simulink model "Compare_3level"  (R2024b)
settings: Solver=ode1  StartTime=0.0  StopTime=4  FixedStep=Ts  RelTol=1e-3
PreLoadFcn:
  | Net_improve_init;L=Lac_MV;Ts=20e-6;Tctrl=Ts;Rac_MV=1;
PostLoadFcn:
  | Net_improve_init;L=Lac_MV;Ts=20e-6;Tctrl=Ts;Rac_MV=1;
InitFcn:
  | Net_improve_init;L=Lac_MV;Ts=20e-6;Tctrl=Ts;Rac_MV=1;
undefined symbols (not defined in the file or in its folder): C1, dend, DiscIntNeverNeededParam, f_cari, fs, Lac_MV, numd, Pref, R1, Vac_peak_MV, Vdc
libraries: powerlib_extras x15, spsControlledVoltageSourceLib x14, spsIGBTDiodeLib x12, spsCurrentMeasurementLib x8, spsGroundLib x7, spsSeriesRLCBranchLib x7, spsVoltageMeasurementLib x6, spsThreePhaseVIMeasurementLib x5, spsControlledCurrentSourceLib x3, spsIdealSwitchLib x3, spsPower3phInstantaneousLib x3, simulink x3
(part 1 of 2)
Description:
  | The Model initialization function Callback automatically
  | 
  | sets the sample time  to 2e-6 sec.  and loads the initial
  | 
  | states vector xInitial. The initial state vector is saved in the
  | 
  | power_acdrive_init.mat file.
  | 
  | 
  | 
  | Check  the Initial state checkbox in the Simulation
  | 
  | parameters/Workspace I/O to start in steady state with a
  | 
  | speed of 120 rad/s and a torque of 0 N.m/s,
  | 
  | 
  | Copyright 2008-2015 The MathWorks, Inc.
settings Model: Creator=WeiLi  LastModifiedBy=KeXing
settings SolverCC: AlgebraicLoopSolver=TrustRegion
settings DataIOCC: SaveFinalState=on  SaveFormat=Array  SignalLoggingSaveFormat=ModelDataLogs  SaveOutput=off  SaveTime=off  ReturnWorkspaceOutputs=off  SignalLoggingName=sigsOut
settings OptimizationCC: BlockReduction=off  ExpressionDepthLimit=2147483647  InitFltsAndDblsToZero=on  LifeSpan=inf
settings DebuggingCC: SaveWithParameterizedLinksMsg=none  UnderspecifiedInitializationDetection=Classic  MergeDetectMultiDrivingBlocksExec=none  CheckExecutionContextPreStartOutputMsg=on  SignalResolutionControl=TryResolveAllWithWarning  MultiTaskDSMMsg=warning  MultiTaskCondExecSysMsg=none  FcnCallInpInsideContextMsg=warning  UnconnectedInputMsg=warning  UnconnectedLineMsg=warning  StateNameClashWarn=warning  SFUnexpectedBacktrackingDiag=warning  SFNoUnconditionalDefaultTransitionDiag=warning  SFExecutionAtInitializationDiag=none  ArithmeticOperatorsInVariantConditions=warning
settings HardwareCC: ProdBitPerPointer=32  ProdBitPerSizeT=32  ProdBitPerPtrDiffT=32  ProdLargestAtomicFloat=None  ProdIntDivRoundTo=Undefined  ProdEndianess=Unspecified  ProdWordSize=32  ProdHWDeviceType=32-bit Generic  TargetUnknown=on
settings ModelReferenceCC: EnableRefExpFcnMdlSchedulingChecks=on  PropagateSignalLabelsOutOfModel=off
settings SFSimCC: SimUseLocalCustomCode=off  CustomCodeUndefinedFunction=UseInterfaceOnly
settings RTWCC: RTWUseLocalCustomCode=off  GPUComputeCapability=3.5
settings CodeAppCC: StateflowObjectComments=on
settings GRTTargetCC: TargetFcnLib=ansi_tfl_tmw.mat  TargetLangStandard=C89/C90 (ANSI)  CombineOutputUpdateFcns=off  GRTInterface=on
settings ConfigComp: CovMetricSettings=dw  CovSaveCumulativeToWorkspaceVar=on  CovSaveSingleToWorkspaceVar=on  CovExternalEMLEnable=off
settings SimscapeCC: SimscapeNormalizeSystem=off

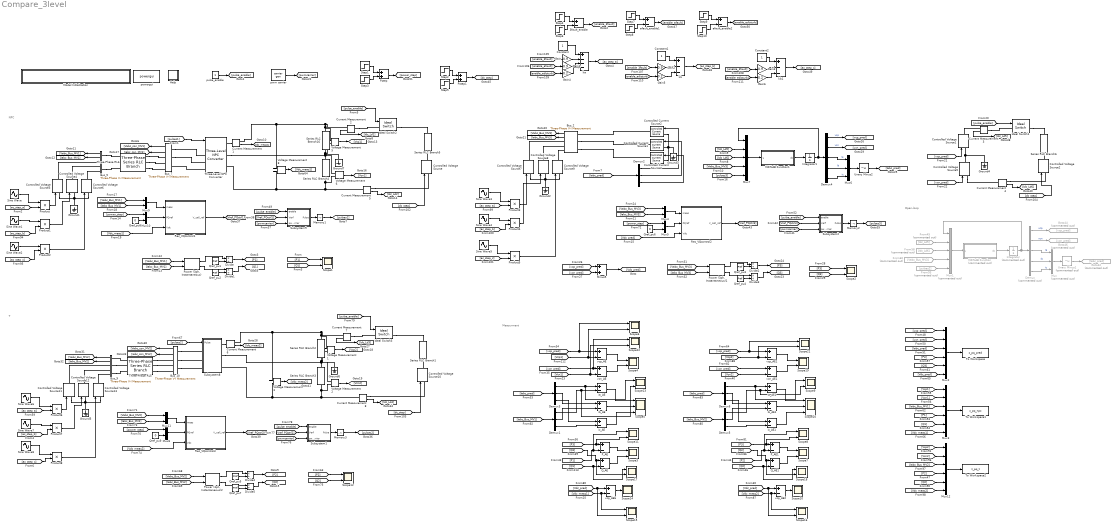
== system Compare_3level ==
  note: NPC
  note: T
  note: Open-loop
  note: Measurment
  3fault_enable : Sum  Inputs=+-
  Bus_{2,5,7,9..10} (5 alike) : spsThreePhaseVIMeasurementLib/Three-Phase V-I Measurement  VoltageMeasurement=phase-to-ground  SetLabelV=off  LabelV=Vabc  Vpu=off  VpuLL=off  CurrentMeasurement=yes  SetLabelI=off  LabelI=Iabc  Ipu=off  Pbase=P_AC  Vbase=V_AC_prim  OutputType=Complex  PhasorSimulation=off  PSBequivalent=0
  Constant : Constant
  Constant1 : Constant
  Constant2 : Constant
  Controlled Current Source1 : spsControlledCurrentSourceLib/Controlled Current Source  Initialize=on  Source_Type=AC  Amplitude=0  Phase=0  Frequency=0  Measurements=None
  Controlled Current Source2 : spsControlledCurrentSourceLib/Controlled Current Source  Initialize=on  Source_Type=AC  Amplitude=0  Phase=0  Frequency=0  Measurements=None
  Controlled Current Source3 : spsControlledCurrentSourceLib/Controlled Current Source  Initialize=on  Source_Type=AC  Amplitude=0  Phase=0  Frequency=0  Measurements=None
  Controlled Voltage Source{,1..2,5,10} (5 alike) : spsControlledVoltageSourceLib/Controlled Voltage Source  Initialize=on  Source_Type=DC  Amplitude=3000  Phase=0  Frequency=0  Measurements=None
  Controlled Voltage Source{3..4,6..9,11..13} (9 alike) : spsControlledVoltageSourceLib/Controlled Voltage Source  Initialize=off  Source_Type=AC  Amplitude=0  Phase=0  Frequency=fs  Measurements=None
  Current Measurement{1..8} (8 alike) : spsCurrentMeasurementLib/Current Measurement  PhasorSimulation=off  OutputType=Complex  PSBequivalent=0
  Demux : Demux  Commented=on  Outputs=5
  Demux{1..3,5..6} (5 alike) : Demux  Outputs=3
  Demux4 : Demux  Outputs=5
  Divide{,1..5} (6 alike) : Product  Inputs=*/
  From45 : From  Commented=on  GotoTag=Idc_Ld5
  From58 : From  Commented=on  GotoTag=Idc_Ld6
  From60 : From  Commented=on  GotoTag=Vabc_Bus_MV3
  From93 : From  Commented=on  GotoTag=pulses2
  Gain{,1..3} (4 alike) : Gain  Gain=0.9
  Gain4 : Gain  Gain=0.2
  Gain5 : Gain  Gain=0.2
  Gain6 : Gain  Gain=0.2
  Goto42 : Goto  Commented=on  GotoTag=Iabc_pred
  Goto44 : Goto  Commented=on  GotoTag=vcp_pred
  Goto46 : Goto  Commented=on  GotoTag=vcn_pred
  Ground{1..7} (7 alike) : spsGroundLib/Ground  LConnTagsString=a
  Help : Subsystem  mask(OpDoc){docfile=../Help/help.html}
      mask init:
      | %patch([1,1,0,0,.8,1],[.8,0,0,1,1,.8],[.8 .8 .8]);
      | %patch([.15 .78 .78 .15 .15],[.8 .8 .83 .83 .8],[.9 .9 .9]);
      | %patch([.15 .78 .78 .15 .15],[.7 .7 .73 .73 .8],[.9 .9 .9]);
      | %patch([.15 .78 .78 .15 .15],[.6 .6 .63 .63 .6],[.9 .9 .9]);
      | %patch([.15 .78 .78 .15 .15],[.5 .5 .53 .53 .5],[.9 .9 .9]);
      | %patch([.15 .78 .78 .15 .15],[.4 .4 .43 .43 .4],[.9 .9 .9]);
      settings: OpenFcn=OpHelp_cb(gcb);
      mask Display: image(imread('opdoc.bmp'))
  Ideal Switch1 : spsIdealSwitchLib/Ideal Switch  Ron=0.001  Lon=0  IC=0  Rs=1e9  Cs=inf  Measurements=on
  Ideal Switch2 : spsIdealSwitchLib/Ideal Switch  Ron=0.001  Lon=0  IC=0  Rs=1e9  Cs=inf  Measurements=on
  Ideal Switch3 : spsIdealSwitchLib/Ideal Switch  Ron=0.001  Lon=0  IC=0  Rs=1e9  Cs=inf  Measurements=on
  Integrator : Integrator  Commented=on
  Integrator1 : Integrator
  MATLAB Function : MATLAB Function  Commented=on  TreatAsAtomicUnit=on
  MATLAB Function1 : MATLAB Function  TreatAsAtomicUnit=on
  Memory1 : Memory
  Memory2 : Memory
  Memory3 : Memory
  Minus5 : Sum
  Model Initialization : Subsystem  mask(Model Functions){InitFcnX=Net_improve_init;L=Lac_MV;Ts=20e-6;Tctrl=Ts;Rac_MV=1;, prel=on, posl=on, inif=on, strf=off}
      mask prompts: InitFcnX "Initialisation"; prel "Preload Function"; posl "PostLoad Function"; inif "InitFcn"; strf "StartFcn"
      mask init:
      | currentBlock = gcb;
      | root = bdroot(currentBlock);
      | 
      | if ~strcmp(get_param(root,'BlockDiagramType'),'library')
      |     if prel==1
      |         set_param(root, 'PreLoadFcn', InitFcnX);
      |     else
      |         set_param(root, 'PreLoadFcn', '');
      |     end
      |     if inif==1
      |         set_param(root, 'InitFcn', InitFcnX);
      |     else
      |         set_param(root, 'InitFcn', '');
      |     end
      |     if strf==1
      |         set_param(root, 'StartFcn', InitFcnX);
      |     else
      |         set_param(root, 'StartFcn', '');
      |     end
      |     if posl==1
      |         set_param(root, 'PostLoadFcn', InitFcnX);
      |     else
      |         set_param(root, 'PostLoadFcn', '');
      |     end
      | end
      | 
      | pos = get_param(currentBlock, 'Position');
      | width = pos(3) - pos(1); height = pos(4) - pos(2);
      | txt = [ upper(root) '\n' '- InitFcn. . . . . '  get_param(root, 'InitFcn') ];
      settings: CopyFcn=set_param(gcb,'LinkStatus','none')
      mask Display: text(5, height*0.5, txt, 'horizontalAlignment', 'left', 'verticalAlignment', 'middle') ;
  Mux : Mux  Commented=on  Inputs=3
  Mux1 : Mux  Commented=on  Inputs=5
  Mux{4..5,8..11} (6 alike) : Mux  Inputs=2
  Mux12 : Mux  Inputs=6
  Mux2 : Mux  Inputs=6
  Mux3 : Mux  Inputs=6
  Mux6 : Mux  Inputs=3
  Mux7 : Mux  Inputs=5
  P_AE : Sum  Inputs=+-
  P_AE1 : Sum  Inputs=+-
  "Power (3ph, Instantaneous)" : spsPower3phInstantaneousLib/Power (3ph, Instantaneous)
  "Power (3ph, Instantaneous)1" : spsPower3phInstantaneousLib/Power (3ph, Instantaneous)
  "Power (3ph, Instantaneous)2" : spsPower3phInstantaneousLib/Power (3ph, Instantaneous)
  Product{,1..8} (9 alike) : Product
  Pstep : Sum
  Pstep1 : Sum
  Q_AE : Sum  Inputs=+-
  Q_AE1 : Sum  Inputs=+-
  Qref_pu{1..5,7} (6 alike) : Constant  Value=Pref
  Qref_pu6 : Constant  Value=0
  Qref_pu8 : Constant  Value=0
  Qref_pu9 : Constant  Value=0
  Rec_VQcontrol1 : Subsystem  mask(converter controller){cm=off, base=[Pref, Vac_peak_MV*sqrt(3/2), Vdc/2, fs], LRx=[Lac_MV, Rac_MV], LRx_inpu=off, Kd=[0.3  2]*10/6  %was [1 0.1]   ; [0.1  1]*1, Kp=[0.3 1]*1     %was [1 0.1]   ; [0.1  1]*1, Kvdc=[2 10]*1;   %was [0.5 1]*20 for Cdc=320uF, Vabc_lim=[-1 1], limitVdq=1.1, nadv=6, xtrIctrl1=[0.4 10 10 -10], Ts=Tctrl}
      mask prompts: cm "control mode (check VQ/uncheck PQ), only one terminal in VQ mode"; base "base value for power(VA), ac voltage(V), dc voltage to ground(V), and frequenvy(Hz) [Sb, Vb, Vdcb,freq]"; LRx "commutation inductance and resistance [Lx, Rx]"; LRx_inpu "[Lx, Rx] in pu if checked/ SI unchecked"; Kd "Kp Ki for d-axis PI control [kp ki]"; Kp "Kp Ki for q-axis PI control [kp ki]"; Kvdc "Kp Ki for Vdc PI control [kp ki]"; Vabc_lim "output Vabc limit [min max]"; limitVdq "limit for Vd,Vq (pu, default = 1.1)"; nadv "nb of time step to compesate for delay (default=1)"; xtrIctrl1 "[kp, kp, limitmax, limitmin] for current control (default=[0.4, 10, 10, -10])"
      mask help:
      | input 1, 6 dimentions, Vabc, Iabc, (SI)
      | input 2, 2 dimentions, Pref, Qref (PU)
      | input 3, 6 dimentions, Vcap at up arm a, lower arm a, up arm b, lower arm b, up arm c and lower arm c.
      | input 4, 1 dimention, pulse on
      | input 5, 1 dimention
      |
      | power or current directions: to go into grid is positive
      mask init:
      | if cm==0;
      |     x=['PQ\nmode'];
      | else
      |     x=['VQ\nmode'];
      | end
      | 
      | Sb=base(1);            %VA 3phase power base;
      | Vb=base(2);       %V, line-line rms voltage base
      | Ib=Sb/(sqrt(3)*Vb); %A, rms current base
      | Zb=Vb^2/Sb ;        %ohm, impedence base
      | Vdc=base(3);      %V Vdc+ to ground or ground to Vdc- 
      | frq=base(4);
      | 
      | if LRx_inpu
      |     Rxpu=LRx(2);
      |     Lxpu=LRx(1);
      | else
      |     Rxpu=LRx(2)/Zb;
      |     Lxpu=LRx(1)*2*pi*frq/Zb;
      | end;
      | 
      | ks=Vdc*sqrt(3/2)/Vb;     % ma=1/ks for 1pu dc ->1pu ac;
      | 
      | Kp=Kd;
      mask DialogControl ParameterTabVar0 Prompt: parameters
      mask DialogControl ParameterTabVar01 Prompt: advanced
      mask Display: disp (x);
  Rec_VQcontrol2 : Subsystem  mask(converter controller){cm=off, base=[Pref, Vac_peak_MV*sqrt(3/2), Vdc/2, fs], LRx=[Lac_MV, Rac_MV], LRx_inpu=off, Kd=[0.3  2]*10/6  %was [1 0.1]   ; [0.1  1]*1, Kp=[0.3 1]*1     %was [1 0.1]   ; [0.1  1]*1, Kvdc=[2 10]*1;   %was [0.5 1]*20 for Cdc=320uF, Vabc_lim=[-1 1], limitVdq=1.1, nadv=6, xtrIctrl1=[0.4 10 10 -10], Ts=Tctrl}
      mask prompts: cm "control mode (check VQ/uncheck PQ), only one terminal in VQ mode"; base "base value for power(VA), ac voltage(V), dc voltage to ground(V), and frequenvy(Hz) [Sb, Vb, Vdcb,freq]"; LRx "commutation inductance and resistance [Lx, Rx]"; LRx_inpu "[Lx, Rx] in pu if checked/ SI unchecked"; Kd "Kp Ki for d-axis PI control [kp ki]"; Kp "Kp Ki for q-axis PI control [kp ki]"; Kvdc "Kp Ki for Vdc PI control [kp ki]"; Vabc_lim "output Vabc limit [min max]"; limitVdq "limit for Vd,Vq (pu, default = 1.1)"; nadv "nb of time step to compesate for delay (default=1)"; xtrIctrl1 "[kp, kp, limitmax, limitmin] for current control (default=[0.4, 10, 10, -10])"
      mask help:
      | input 1, 6 dimentions, Vabc, Iabc, (SI)
      | input 2, 2 dimentions, Pref, Qref (PU)
      | input 3, 6 dimentions, Vcap at up arm a, lower arm a, up arm b, lower arm b, up arm c and lower arm c.
      | input 4, 1 dimention, pulse on
      | input 5, 1 dimention
      |
      | power or current directions: to go into grid is positive
      mask init: same as Compare_3level/Rec_VQcontrol1
      mask DialogControl ParameterTabVar0 Prompt: parameters
      mask DialogControl ParameterTabVar01 Prompt: advanced
      mask Display: disp (x);
  Rec_VQcontrol3 : Subsystem  mask(converter controller){cm=off, base=[Pref, Vac_peak_MV*sqrt(3/2), Vdc/2, fs], LRx=[Lac_MV, Rac_MV], LRx_inpu=off, Kd=[0.3  2]*10/6  %was [1 0.1]   ; [0.1  1]*1, Kp=[0.3 1]*1     %was [1 0.1]   ; [0.1  1]*1, Kvdc=[2 10]*1;   %was [0.5 1]*20 for Cdc=320uF, Vabc_lim=[-1 1], limitVdq=1.1, nadv=6, xtrIctrl1=[0.4 10 10 -10], Ts=Tctrl}
      mask prompts: cm "control mode (check VQ/uncheck PQ), only one terminal in VQ mode"; base "base value for power(VA), ac voltage(V), dc voltage to ground(V), and frequenvy(Hz) [Sb, Vb, Vdcb,freq]"; LRx "commutation inductance and resistance [Lx, Rx]"; LRx_inpu "[Lx, Rx] in pu if checked/ SI unchecked"; Kd "Kp Ki for d-axis PI control [kp ki]"; Kp "Kp Ki for q-axis PI control [kp ki]"; Kvdc "Kp Ki for Vdc PI control [kp ki]"; Vabc_lim "output Vabc limit [min max]"; limitVdq "limit for Vd,Vq (pu, default = 1.1)"; nadv "nb of time step to compesate for delay (default=1)"; xtrIctrl1 "[kp, kp, limitmax, limitmin] for current control (default=[0.4, 10, 10, -10])"
      mask help:
      | input 1, 6 dimentions, Vabc, Iabc, (SI)
      | input 2, 2 dimentions, Pref, Qref (PU)
      | input 3, 6 dimentions, Vcap at up arm a, lower arm a, up arm b, lower arm b, up arm c and lower arm c.
      | input 4, 1 dimention, pulse on
      | input 5, 1 dimention
      |
      | power or current directions: to go into grid is positive
      mask init: same as Compare_3level/Rec_VQcontrol1
      mask DialogControl ParameterTabVar0 Prompt: parameters
      mask DialogControl ParameterTabVar01 Prompt: advanced
      mask Display: disp (x);
  Scope{1..4,6..9,11..13,15..19,21..22} (18 alike) : Scope  NumInputPorts=2
  Scope10 : Scope
  Scope14 : Scope
  Scope20 : Scope  NumInputPorts=3
  Scope5 : Scope  NumInputPorts=3
  Series RLC Branch1 : spsSeriesRLCBranchLib/Series RLC Branch  LConnTagsString=__new0  RConnTagsString=__new0  BranchType=R  Resistance=3e3^2/(Pref)/10*2  Inductance=1e-3  SetiL0=off  InitialCurrent=0  Capacitance=C1  Setx0=off  InitialVoltage=0  Measurements=None
  Series RLC Branch{2..4,16} (4 alike) : spsSeriesRLCBranchLib/Series RLC Branch  LConnTagsString=__new0  RConnTagsString=__new0  BranchType=C  Resistance=R1  Inductance=1e-3  SetiL0=off  InitialCurrent=0  Capacitance=C1  Setx0=off  InitialVoltage=0  Measurements=None
  Series RLC Branch5 : spsSeriesRLCBranchLib/Series RLC Branch  LConnTagsString=__new0  RConnTagsString=__new0  BranchType=R  Resistance=3e3^2/(Pref)/10*2  Inductance=1e-3  SetiL0=off  InitialCurrent=0  Capacitance=C1  Setx0=off  InitialVoltage=0  Measurements=None
  Series RLC Branch6 : spsSeriesRLCBranchLib/Series RLC Branch  LConnTagsString=__new0  RConnTagsString=__new0  BranchType=R  Resistance=3e3^2/(Pref)/10*2  Inductance=1e-3  SetiL0=off  InitialCurrent=0  Capacitance=C1  Setx0=off  InitialVoltage=0  Measurements=None
  Sine Wave : Sin  Amplitude=3e3/2*sqrt(2/3)  Frequency=2*pi*fs  SampleTime=0
  Sine Wave1 : Sin  Amplitude=3e3/2*sqrt(2/3)  Frequency=2*pi*fs  Phase=-2*pi/3  SampleTime=0
  Sine Wave2 : Sin  Amplitude=3e3/2*sqrt(2/3)  Frequency=2*pi*fs  Phase=+2*pi/3  SampleTime=0
  Sine Wave3 : Sin  Amplitude=3e3/2*sqrt(2/3)  Frequency=2*pi*fs  SampleTime=0
  Sine Wave4 : Sin  Amplitude=3e3/2*sqrt(2/3)  Frequency=2*pi*fs  Phase=-2*pi/3  SampleTime=0
  Sine Wave5 : Sin  Amplitude=3e3/2*sqrt(2/3)  Frequency=2*pi*fs  Phase=+2*pi/3  SampleTime=0
  Sine Wave6 : Sin  Amplitude=3e3/2*sqrt(2/3)  Frequency=2*pi*fs  SampleTime=0
  Sine Wave7 : Sin  Amplitude=3e3/2*sqrt(2/3)  Frequency=2*pi*fs  Phase=-2*pi/3  SampleTime=0
  Sine Wave8 : Sin  Amplitude=3e3/2*sqrt(2/3)  Frequency=2*pi*fs  Phase=+2*pi/3  SampleTime=0
  Step1 : Step  Time=2.75  Before=-0.8  After=-0.6  SampleTime=0
  Step10 : Step  Time=3.85  SampleTime=0
  Step2 : Step  Time=3.25  Before=3000  After=2400  SampleTime=0
  Step3 : Step  Time=3.0  Before=0.0  After=-0.2  SampleTime=0
  Step4 : Step  Time=1.75  SampleTime=0
  Step5 : Step  Time=3.5  After=600  SampleTime=0
  Step6 : Step  Time=1.9  SampleTime=0
  Step7 : Step  Time=2.5  SampleTime=0
  Step8 : Step  Time=2.65  SampleTime=0
  Step9 : Step  Time=3.70  SampleTime=0
  Subsystem1 : Subsystem
  Subsystem2 : Subsystem
  Subsystem8 : Subsystem
  Subsystem9 : Subsystem
  Three-Level NPC Converter : spsThreeLevelNPCConverterLib/Three-Level NPC Converter  ModelType=Switching devices  Ron=IGBT_Ron  Rs=1e5  Cs=IGBT_Cs  Vforward=[0,0]  Ron_Diode=1e-3  Rs_Diode=1e6  Cs_Diode=inf  Vf_Diode=1e-3  Rs_CurrentSource=inf  Ron_ACsource=1e-3
      settings: LibrarySourceBlock=|
      | sps_lib/Power Electronics/Three-Level
      | NPC Converter
  Three-Phase RL3 : spsThreePhaseSeriesRLCBranchLib/Three-Phase Series RLC Branch  LConnTagsString=A|B|C  RConnTagsString=A|B|C  BranchType=RL  Resistance=Rac_MV  Inductance=Lac_MV  Capacitance=1e-6  Measurements=None
  Three-Phase RL5 : spsThreePhaseSeriesRLCBranchLib/Three-Phase Series RLC Branch  LConnTagsString=A|B|C  RConnTagsString=A|B|C  BranchType=RL  Resistance=Rac_MV  Inductance=Lac_MV  Capacitance=1e-6  Measurements=None
  To Workspace : ToWorkspace  VariableName=z_pq_pred  SampleTime=-1
      settings: Save2DSignal=2-D array (concatenate along first dimension)
  To Workspace1 : ToWorkspace  VariableName=z_pq_npc  SampleTime=-1
      settings: Save2DSignal=2-D array (concatenate along first dimension)
  To Workspace2 : ToWorkspace  VariableName=z_pq_t  SampleTime=-1
      settings: Save2DSignal=2-D array (concatenate along first dimension)
  Unary Minus1 : UnaryMinus  Commented=on
  Unary Minus2 : UnaryMinus
  Voltage Measurement{1..3,5..6,8} (6 alike) : spsVoltageMeasurementLib/Voltage Measurement  PhasorSimulation=off  OutputType=Complex  PSBequivalent=0
  afault_enable1 : Sum  Inputs=+-
  afault_enable2 : Sum  Inputs=+-
  ia_AE : Sum  Inputs=+-
  ia_AE1 : Sum  Inputs=+-
  ib_AE : Sum  Inputs=+-
  ib_AE1 : Sum  Inputs=+-
  ic_AE : Sum  Inputs=+-
  ic_AE1 : Sum  Inputs=+-
  ka : Sum  Inputs=+---
  kb : Sum  Inputs=+--
  kb1 : Sum  Inputs=+--
  powergui : spspowerguiLib/powergui  Priority=2  SimulationMode=Discrete  SampleTime=Ts  frequency=60  Iterations=50  frequencyindice=0  Pbase=100e6  ErrMax=1e-4  UnitsV=kV  UnitsW=MW  buscounter=0  FunctionMessages=off  echomessages=off  EnableUseOfTLC=off  CurrentSourceSwitches=off  DisableSnubberDevices=off  DisableRonSwitches=off  DisableVfSwitches=off  DisplayEquations=off  AutomaticDiscreteSolvers=off  SolverType=Backward Euler  Interpol=off  ExternalGateDelay=off  methode=off  Ts=0  x0status=blocks  SPID=off  SwTol=0  HookPort=off  NonlinearTolerance=1e-4  nMaxIteration=100  ContinueOnMaxIteration=off  RestoreLinks=warning  ResistiveCurrentMeasurement=off  Frange=[0:2:500]  Ylog=off  Xlog=on  ShowGrid=off  save=off  variable=ZData  structure=VI  ZoomFFT=off  StartTime=9  cycles=10  DisplayStyle=2  fundamental=300/pi  FreqAxis=off  MaxFrequency=1000  frequencyindicesteady=1  RmsSteady=1  display=off
  pulse_enable : Constant
  pwm carrier : libMMCcpuv2/carrier gen  fc=f_cari*2  range=[1 0]  Ms=3  Ns=1
  vcn_AE : Sum  Inputs=+-
  vcn_AE1 : Sum  Inputs=+-
  vcp_AE{,1..2,6} (4 alike) : Sum  Inputs=+-
  wires:
  Bus_7/1 -> [Vabc_con_MV1]
  Bus_5/1 -> [Vabc_Bus_MV1]
  Bus_5/2 -> [Iabc_Bus_MV1]
  [pulses1] -> Three-Level NPC Converter/1
  [pulses2] -> Subsystem8/1(Pulse)
  Bus_9/1 -> [Vabc_Bus_MV2]
  Bus_9/2 -> [Iabc_Bus_MV2]
  Bus_10/1 -> [Vabc_con_MV2]
  pwm carrier/1 -> [pwmcarrier]
  pulse_enable/1 -> [pulse_enable]
  [ac_step_c] -> Product2/2
  Sine Wave1/1 -> Product1/1
  [ac_step_a] -> Product/2
  Product2/1 -> Controlled Voltage Source6/1
  Product/1 -> Controlled Voltage Source3/1
  Sine Wave/1 -> Product/1
  Sine Wave2/1 -> Product2/1
  Product1/1 -> Controlled Voltage Source4/1
  [ac_step_b] -> Product1/2
  Bus_7/2 -> [iabc_con_MV1]
  [pwmcarrier] -> Subsystem9/3(pwmcarrier)
  [Iabc_Bus_MV1] -> Mux9/2
  [Vabc_Bus_MV1] -> "Power (3ph, Instantaneous)"/1
  [P1] -> Scope1/1
  [Vref_PQctrl1] -> Subsystem9/2(Verf)
  [Vdc_meas1] -> Rec_VQcontrol1/3(Vdc)
  Qref_pu8/1 -> Mux10/2
  Qref_pu1/1 -> Divide/2
  [Vabc_Bus_MV1] -> Mux9/1
  Mux9/1 -> Rec_VQcontrol1/1(meas)
  [pulse_enable] -> Subsystem9/1(enable)
  [power_step] -> Mux10/1
  Subsystem9/1(Pulse) -> Memory1/1
  Rec_VQcontrol1/1(V_cell_ref) -> [Vref_PQctrl1]
  Divide/1 -> [P1]
  Qref_pu2/1 -> Divide1/2
  Mux10/1 -> Rec_VQcontrol1/2(PQref)
  [Iabc_Bus_MV1] -> "Power (3ph, Instantaneous)"/2
  Divide1/1 -> [Q1]
  "Power (3ph, Instantaneous)"/2 -> Divide1/1
  [Q1] -> Scope1/2
  Memory1/1 -> [pulses1]
  "Power (3ph, Instantaneous)"/1 -> Divide/1
  Voltage Measurement8/1 -> [Vdc_meas1]
  Current Measurement2/1 -> [Idc_Ld1]
  Voltage Measurement6/1 -> [Vcn1]
  Current Measurement5/1 -> [Idc_Ld2]
  [pulse_enable] -> Ideal Switch2/1
  [dc_step] -> Controlled Voltage Source/1
  Current Measurement1/1 -> [Idc_meas1]
  Voltage Measurement5/1 -> [Vcp1]
  [ac_step_b] -> Product7/2
  Sine Wave7/1 -> Product7/1
  Product7/1 -> Controlled Voltage Source12/1
  Sine Wave6/1 -> Product6/1
  Sine Wave8/1 -> Product8/1
  [ac_step_a] -> Product6/2
  [ac_step_c] -> Product8/2
  Product8/1 -> Controlled Voltage Source13/1
  Product6/1 -> Controlled Voltage Source11/1
  Bus_10/2 -> [iabc_con_MV2]
  [power_step] -> Mux8/1
  "Power (3ph, Instantaneous)2"/2 -> Divide5/1
  Qref_pu9/1 -> Mux8/2
  [Vabc_Bus_MV2] -> "Power (3ph, Instantaneous)2"/1
  [Iabc_Bus_MV2] -> "Power (3ph, Instantaneous)2"/2
  Subsystem1/1(Pulse) -> Memory3/1
  [Iabc_Bus_MV2] -> Mux11/2
  Memory3/1 -> [pulses2]
  Qref_pu5/1 -> Divide4/2
  Rec_VQcontrol3/1(V_cell_ref) -> [Vref_PQctrl2]
  Qref_pu7/1 -> Divide5/2
  [Vabc_Bus_MV2] -> Mux11/1
  [pwmcarrier] -> Subsystem1/3(pwmcarrier)
  [pulse_enable] -> Subsystem1/1(enable)
  "Power (3ph, Instantaneous)2"/1 -> Divide4/1
  Divide4/1 -> [P2]
  [Q2] -> Scope12/2
  Mux11/1 -> Rec_VQcontrol3/1(meas)
  [Vref_PQctrl2] -> Subsystem1/2(Verf)
  Mux8/1 -> Rec_VQcontrol3/2(PQref)
  Divide5/1 -> [Q2]
  [P2] -> Scope12/1
  [Vdc_meas2] -> Rec_VQcontrol3/3(Vdc)
  Voltage Measurement2/1 -> [Vcn2]
  Current Measurement6/1 -> [Idc_meas2]
  Current Measurement8/1 -> [Idc_Ld4]
  Current Measurement7/1 -> [Idc_Ld3]
  [dc_step] -> Controlled Voltage Source10/1
  Voltage Measurement1/1 -> [Vcp2]
  Voltage Measurement3/1 -> [Vdc_meas2]
  [pulse_enable] -> Ideal Switch3/1
  [enable_afault] -> Gain1/1
  [enable_edisturb] -> Gain4/1
  Step7/1 -> afault_enable1/1
  afault_enable2/1 -> [enable_edisturb]
  Step5/1 -> Pstep1/2
  Constant/1 -> ka/1
  Gain4/1 -> ka/4
  Gain3/1 -> kb1/2
  Step3/1 -> Pstep/2
  Step6/1 -> 3fault_enable/2
  kb/1 -> [ac_step_b]
  Pstep1/1 -> [dc_step]
  Step10/1 -> afault_enable2/2
  Step4/1 -> 3fault_enable/1
  afault_enable1/1 -> [enable_afault]
  [enable_3fault] -> Gain/1
  Gain6/1 -> kb1/3
  ka/1 -> [ac_step_a]
  Gain1/1 -> ka/3
  [enable_edisturb] -> Gain5/1
  kb1/1 -> [ac_step_c]
  Gain5/1 -> kb/3
  Step2/1 -> Pstep1/1
  [enable_3fault] -> Gain3/1
  Gain2/1 -> kb/2
  3fault_enable/1 -> [enable_3fault]
  Constant1/1 -> kb/1
  [enable_edisturb] -> Gain6/1
  Step9/1 -> afault_enable2/1
  Step8/1 -> afault_enable1/2
  Constant2/1 -> kb1/1
  Step1/1 -> Pstep/1
  Gain/1 -> ka/2
  Pstep/1 -> [power_step]
  [enable_3fault] -> Gain2/1
  [Iabc_pred] -> Demux2/1
  Bus_2/2 -> [Iabc_Bus_MV3]
  Product3/1 -> Controlled Voltage Source7/1
  Demux2/2 -> Controlled Current Source1/1
  [vcp_pred] -> Minus5/1
  Sine Wave3/1 -> Product3/1
  Minus5/1 -> [Vdc_pred]
  [ac_step_a] -> Product3/2
  Sine Wave4/1 -> Product4/1
  Demux2/1 -> Controlled Current Source2/1
  Demux2/3 -> Controlled Current Source3/1
  Sine Wave5/1 -> Product5/1
  Product5/1 -> Controlled Voltage Source9/1
  [ac_step_b] -> Product4/2
  [vcn_pred] -> Minus5/2
  Bus_2/1 -> [Vabc_Bus_MV3]
  [ac_step_c] -> Product5/2
  Product4/1 -> Controlled Voltage Source8/1
  Qref_pu4/1 -> Divide3/2
  "Power (3ph, Instantaneous)1"/1 -> Divide2/1
  [Iabc_Bus_MV3] -> "Power (3ph, Instantaneous)1"/2
  Divide2/1 -> [P3]
  "Power (3ph, Instantaneous)1"/2 -> Divide3/1
  Divide3/1 -> [Q3]
  [Vabc_Bus_MV3] -> "Power (3ph, Instantaneous)1"/1
  Qref_pu3/1 -> Divide2/2
  [Vdc_pred] -> Rec_VQcontrol2/3(Vdc)
  Rec_VQcontrol2/1(V_cell_ref) -> [Vref_PQctrl3]
  [Iabc_Bus_MV3] -> Mux4/2
  Mux5/1 -> Rec_VQcontrol2/2(PQref)
  Qref_pu6/1 -> Mux5/2
  [power_step] -> Mux5/1
  Mux4/1 -> Rec_VQcontrol2/1(meas)
  [Vabc_Bus_MV3] -> Mux4/1
  [Vref_PQctrl3] -> Subsystem2/2(Verf)
  [pulse_enable] -> Subsystem2/1(enable)
  [pwmcarrier] -> Subsystem2/3(pwmcarrier)
  Memory2/1 -> [pulses3]
  Subsystem2/1(Pulse) -> Memory2/1
  Demux4/4 -> Mux6/2  "ib"
  Demux4/5 -> Mux6/3  "ic"
  [Vabc_Bus_MV3] -> Mux7/4
  Mux7/1 -> MATLAB Function1/1(u)
  Demux4/2 -> [vcn_pred]  "vcn"
  [pulses3] -> Mux7/5
  Mux6/1 -> Unary Minus2/1
  [Idc_Ld6] -> Mux7/3
  Demux4/3 -> Mux6/1  "ia"
  Integrator1/1 -> Mux7/1, Demux4/1
  Demux4/1 -> [vcp_pred]  "vcp"
  Unary Minus2/1 -> [Iabc_pred]
  [Idc_Ld5] -> Mux7/2
  MATLAB Function1/1(dz) -> Integrator1/1
  Current Measurement3/1 -> [Idc_Ld5]
  [pulse_enable] -> Ideal Switch1/1
  Current Measurement4/1 -> [Idc_Ld6]
  [vcn_pred] -> Controlled Voltage Source5/1
  [vcp_pred] -> Controlled Voltage Source1/1
  [dc_step] -> Controlled Voltage Source2/1
  Demux/5 -> Mux/3  "ic"
  Demux/1 -> Goto44/1  "vcp"
  Demux/4 -> Mux/2  "ib"
  MATLAB Function/1(dz) -> Integrator/1
  From60/1 -> Mux1/4
  Mux1/1 -> MATLAB Function/1(u)
  From93/1 -> Mux1/5
  Demux/2 -> Goto46/1  "vcn"
  From58/1 -> Mux1/3
  Integrator/1 -> Mux1/1, Demux/1
  Demux/3 -> Mux/1  "ia"
  Mux/1 -> Unary Minus1/1
  Unary Minus1/1 -> Goto42/1
  From45/1 -> Mux1/2
  [Q3] -> Scope2/2
  [P3] -> Scope2/1
  [Vdc_meas2] -> Scope16/1, vcp_AE2/2
  [vcp_pred] -> Mux2/1
  vcn_AE/1 -> Scope4/2
  [Vcp2] -> Scope21/2, vcp_AE1/2
  [Q3] -> Scope18/2, Q_AE1/1
  [Iabc_Bus_MV2] -> Demux5/1
  [Q2] -> Scope18/1, Q_AE1/2
  [Vdc_pred] -> Scope15/2, vcp_AE6/1
  [Vcp1] -> Scope6/2, vcp_AE/2
  vcp_AE/1 -> Scope4/1
  vcp_AE1/1 -> Scope19/1
  Q_AE1/1 -> Scope7/2
  [vcn_pred] -> Mux2/2
  [P3] -> Mux2/4
  Demux1/3 -> ic_AE/2
  P_AE1/1 -> Scope7/1
  Demux6/1 -> Scope9/1, ia_AE1/1
  [Vdc_meas2] -> Mux12/6
  ia_AE/1 -> Scope5/1
  Demux6/2 -> ib_AE1/1
  [vcn_pred] -> vcn_AE1/1
  ia_AE1/1 -> Scope20/1
  Mux3/1 -> To Workspace1/1
  [Q1] -> Scope17/1, Q_AE/2
  ib_AE1/1 -> Scope20/2
  [P3] -> Scope11/2, P_AE/1
  [vcp_pred] -> Scope21/1, vcp_AE1/1
  ic_AE/1 -> Scope5/3
  Mux2/1 -> To Workspace/1
  [Vdc_meas1] -> Scope15/1, vcp_AE6/2
  [Vdc_pred] -> Scope16/2, vcp_AE2/1
  vcn_AE1/1 -> Scope19/2
  [Vcp2] -> Mux12/1
  [Vcn2] -> Mux12/2
  [Vdc_meas1] -> Mux3/6
  Demux5/3 -> ic_AE1/2
  Mux12/1 -> To Workspace2/1
  Demux1/2 -> ib_AE/2
  [Iabc_Bus_MV1] -> Demux1/1
  vcp_AE6/1 -> Scope14/1
  [Iabc_pred] -> Mux2/3
  [Vcn1] -> Scope22/2, vcn_AE/2
  ic_AE1/1 -> Scope20/3
  Demux3/1 -> Scope13/1, ia_AE/1
  [P2] -> P_AE1/2, Scope8/1
  [P2] -> Mux12/4
  [Vcn2] -> vcn_AE1/2
  [P1] -> P_AE/2, Scope11/1
  Q_AE/1 -> Scope3/2
  [Q2] -> Mux12/5
  [Iabc_Bus_MV1] -> Mux3/3
  [P3] -> Scope8/2, P_AE1/1
  Demux3/2 -> ib_AE/1
  [vcn_pred] -> Scope22/1, vcn_AE/1
  [vcp_pred] -> Scope6/1, vcp_AE/1
  Demux1/1 -> Scope13/2, ia_AE/2
  ib_AE/1 -> Scope5/2
  [Vcn1] -> Mux3/2
  Demux3/3 -> ic_AE/1
  [P1] -> Mux3/4
  vcp_AE2/1 -> Scope10/1
  [Q1] -> Mux3/5
  Demux5/1 -> Scope9/2, ia_AE1/2
  [Iabc_pred] -> Demux3/1
  [Q3] -> Scope17/2, Q_AE/1
  P_AE/1 -> Scope3/1
  [Vdc_pred] -> Mux2/6
  [Iabc_Bus_MV2] -> Mux12/3
  [Q3] -> Mux2/5
  [Vcp1] -> Mux3/1
  [Iabc_pred] -> Demux6/1
  Demux6/3 -> ic_AE1/1
  Demux5/2 -> ib_AE1/2
  connections:
  Bus_7/LConn1 -- Three-Level NPC Converter/LConn1
  Bus_7/LConn2 -- Three-Level NPC Converter/LConn2
  Three-Level NPC Converter/LConn3 -- Bus_7/LConn3
  Three-Phase RL3/RConn1 -- Bus_7/RConn1
  Three-Phase RL3/RConn2 -- Bus_7/RConn2
  Three-Phase RL3/RConn3 -- Bus_7/RConn3
  Bus_5/LConn2 -- Three-Phase RL3/LConn2
  Bus_5/LConn1 -- Three-Phase RL3/LConn1
  Bus_5/LConn3 -- Three-Phase RL3/LConn3
  Bus_9/LConn2 -- Three-Phase RL5/LConn2
  Three-Phase RL5/LConn1 -- Bus_9/LConn1
  Bus_9/LConn3 -- Three-Phase RL5/LConn3
  Bus_10/LConn2 -- Subsystem8/LConn2
  Bus_10/LConn1 -- Subsystem8/LConn1
  Bus_10/LConn3 -- Subsystem8/LConn3
  Three-Phase RL5/RConn1 -- Bus_10/RConn1
  Three-Phase RL5/RConn2 -- Bus_10/RConn2
  Three-Phase RL5/RConn3 -- Bus_10/RConn3
  Controlled Voltage Source4/LConn1 -- Controlled Voltage Source6/LConn1 -- Controlled Voltage Source3/LConn1 -- Ground1/LConn1
  Bus_5/RConn3 -- Controlled Voltage Source6/RConn1
  Bus_5/RConn1 -- Controlled Voltage Source3/RConn1
  Bus_5/RConn2 -- Controlled Voltage Source4/RConn1
  Current Measurement1/RConn1 -- Voltage Measurement8/LConn1 -- Voltage Measurement5/LConn1 -- Series RLC Branch16/LConn1 -- Current Measurement2/RConn1
  Series RLC Branch16/RConn1 -- Three-Level NPC Converter/RConn2 -- Series RLC Branch4/LConn1 -- Voltage Measurement6/LConn1 -- Ground7/LConn1 -- Voltage Measurement5/LConn2
  Voltage Measurement8/LConn2 -- Series RLC Branch4/RConn1 -- Voltage Measurement6/LConn2 -- Current Measurement5/LConn1 -- Three-Level NPC Converter/RConn3
  Current Measurement2/LConn1 -- Ideal Switch2/LConn1
  Three-Level NPC Converter/RConn1 -- Current Measurement1/LConn1
  Current Measurement5/RConn1 -- Controlled Voltage Source/LConn1
  Controlled Voltage Source/RConn1 -- Series RLC Branch5/LConn1
  Ideal Switch2/RConn1 -- Series RLC Branch5/RConn1
  Controlled Voltage Source11/LConn1 -- Controlled Voltage Source12/LConn1 -- Ground5/LConn1 -- Controlled Voltage Source13/LConn1
  Bus_9/RConn3 -- Controlled Voltage Source13/RConn1
  Bus_9/RConn1 -- Controlled Voltage Source11/RConn1
  Bus_9/RConn2 -- Controlled Voltage Source12/RConn1
  Current Measurement6/RConn1 -- Series RLC Branch2/LConn1 -- Voltage Measurement1/LConn1 -- Current Measurement7/RConn1 -- Voltage Measurement3/LConn1
  Voltage Measurement2/LConn1 -- Series RLC Branch3/LConn1 -- Subsystem8/RConn2 -- Ground6/LConn1 -- Series RLC Branch2/RConn1 -- Voltage Measurement1/LConn2
  Voltage Measurement2/LConn2 -- Series RLC Branch3/RConn1 -- Current Measurement8/LConn1 -- Subsystem8/RConn3 -- Voltage Measurement3/LConn2
  Ideal Switch3/RConn1 -- Series RLC Branch1/RConn1
  Controlled Voltage Source10/RConn1 -- Series RLC Branch1/LConn1
  Subsystem8/RConn1 -- Current Measurement6/LConn1
  Current Measurement7/LConn1 -- Ideal Switch3/LConn1
  Current Measurement8/RConn1 -- Controlled Voltage Source10/LConn1
  Controlled Voltage Source8/LConn1 -- Ground2/LConn1 -- Controlled Voltage Source9/LConn1 -- Controlled Voltage Source7/LConn1
  Bus_2/RConn2 -- Controlled Voltage Source8/RConn1
  Controlled Current Source2/RConn1 -- Bus_2/LConn1
  Bus_2/RConn3 -- Controlled Voltage Source9/RConn1
  Bus_2/RConn1 -- Controlled Voltage Source7/RConn1
  Bus_2/LConn3 -- Controlled Current Source3/RConn1
  Bus_2/LConn2 -- Controlled Current Source1/RConn1
  Controlled Current Source2/LConn1 -- Ground3/LConn1 -- Controlled Current Source3/LConn1 -- Controlled Current Source1/LConn1
  Controlled Voltage Source1/LConn1 -- Controlled Voltage Source5/RConn1 -- Ground4/LConn1
  Current Measurement3/RConn1 -- Controlled Voltage Source1/RConn1
  Controlled Voltage Source5/LConn1 -- Current Measurement4/LConn1
  Ideal Switch1/RConn1 -- Series RLC Branch6/RConn1
  Controlled Voltage Source2/RConn1 -- Series RLC Branch6/LConn1
  Current Measurement4/RConn1 -- Controlled Voltage Source2/LConn1
  Current Measurement3/LConn1 -- Ideal Switch1/LConn1

== system Compare_3level/Help ==

== system Compare_3level/Model Initialization ==

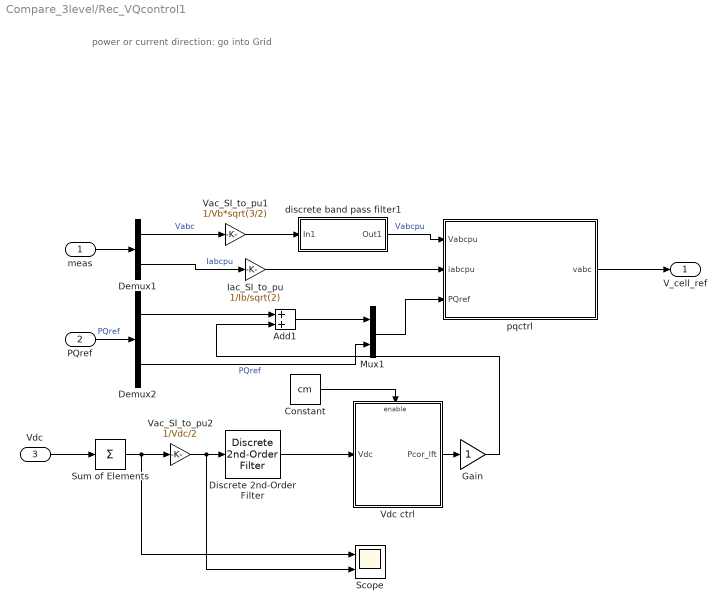
== system Compare_3level/Rec_VQcontrol1 ==
  note: power or current direction: go into Grid
  meas : Inport
  PQref : Inport  Port=2
  Vdc : Inport  Port=3
  Add1 : Sum
  Constant : Constant  Value=cm
  Demux1 : Demux  Outputs=[3 3 ]
  Demux2 : Demux  Outputs=2
  Discrete 2nd-Order Filter : powerlib_extras/Discrete  Control Blocks/Discrete  2nd-Order Filter  FilterType=Lowpass  Fo=90  Zeta=0.707  Ts=Ts  Initialize=off  Vac_Init=[0.8 -25 60]  Vdc_Init=-0.4  PlotResponse=off  param1=[1 500 1]
  Gain : Gain
  Iac_SI_to_pu : Gain  Gain=1/Ib/sqrt(2)
  Mux1 : Mux  Inputs=2
  Scope : Scope  NumInputPorts=2
  Sum of Elements : Sum  Inputs=+
  Vac_SI_to_pu1 : Gain  Gain=1/Vb*sqrt(3/2)
  Vac_SI_to_pu2 : Gain  Gain=1/Vdc/2  SampleTime=Ts
  Vdc ctrl : Subsystem
  discrete band pass filter1 : Subsystem  mask(discrete transfer Fcn generator){Fo=frq, adj1=1, inistate=0, Ts=Ts, bodedw=off}
      mask prompts: Fo "F0 (Hz)"; adj1 "adj (1 for no adjustment, larger adj for wider band pass)"; inistate "Initial states"; Ts "Sample time (must be explicite)"; bodedw "draw Bode diagram of filter"
      mask help:
      | This block transfer a continous TF to a discrete TF
      | using Bilinear (Tustin) approximation
      mask init:
      | AD1=tf([1 0],1);
      | 
      | %second order
      | % Fo=50; %cut off freq.
      | % omega0=Fo*2*pi;
      | % adj1=3;   %adjustment 1
      | Zeta= 0.707*adj1; %Damping factor Zeta ( Q = 1 / (2*Zeta) ):
      | Wo=2*pi*Fo;
      | % str=sprintf(' Fo=%iHz\n\n',Fo);
      |  n2=0; n1=0;n0=Wo*Wo;
      |  d2=1;d1=2*Zeta*Wo;d0=Wo*Wo;
      | numc=[n2 n1 n0];
      | denc=[d2 d1 d0];
      | AD3=tf(numc,denc);
      | 
      | AD4=AD1*AD3;
      | [mag1,pha1]=bode(AD4,Wo);
      | mag0=mag1;
      | AD=AD4/mag0;
      | 
      | if bodedw==1
      |     figure;
      |     h=bodeplot(AD1,AD3,AD);
      |     setoptions(h,'FreqUnits','Hz');
      |     grid on;
      |     title(['Bode Diagram, adj=',num2str(adj1)]);
      | end;
      |     
      | % gg=tf(num,den);
      | ggd=c2d(AD,Ts,'tustin');
      | [numd,dend] = tfdata(ggd,'v');
  pqctrl : Subsystem
  V_cell_ref : Outport  VectorParamsAs1DForOutWhenUnconnected=off
  wires:
  Constant/1 -> Vdc ctrl/Enable
  Vac_SI_to_pu1/1 -> discrete band pass filter1/1(In1)
  Vac_SI_to_pu2/1 -> Scope/2, Discrete 2nd-Order Filter/1
  Vdc/1 -> Sum of Elements/1
  Discrete 2nd-Order Filter/1 -> Vdc ctrl/1(Vdc)
  Mux1/1 -> pqctrl/3(PQref)
  Demux2/2 -> Mux1/2  "PQref"
  Add1/1 -> Mux1/1
  Vdc ctrl/1(Pcor_lft) -> Gain/1
  Demux2/1 -> Add1/1
  Iac_SI_to_pu/1 -> pqctrl/2(iabcpu)
  Demux1/1 -> Vac_SI_to_pu1/1  "Vabc"
  Demux1/2 -> Iac_SI_to_pu/1  "Iabcpu"
  meas/1 -> Demux1/1
  discrete band pass filter1/1(Out1) -> pqctrl/1(Vabcpu)  "Vabcpu"
  PQref/1 -> Demux2/1  "PQref"
  pqctrl/1(vabc) -> V_cell_ref/1
  Sum of Elements/1 -> Scope/1, Vac_SI_to_pu2/1
  Gain/1 -> Add1/2

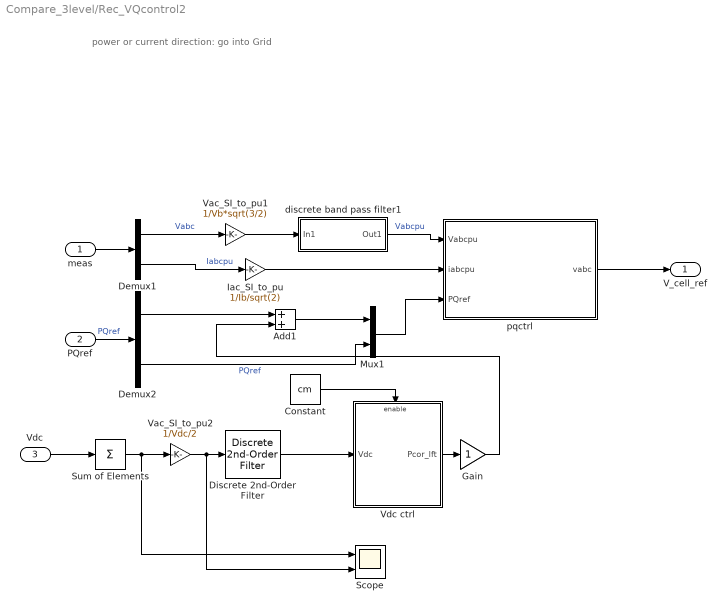
== system Compare_3level/Rec_VQcontrol2 ==
  note: power or current direction: go into Grid
  meas : Inport
  PQref : Inport  Port=2
  Vdc : Inport  Port=3
  Add1 : Sum
  Constant : Constant  Value=cm
  Demux1 : Demux  Outputs=[3 3 ]
  Demux2 : Demux  Outputs=2
  Discrete 2nd-Order Filter : powerlib_extras/Discrete  Control Blocks/Discrete  2nd-Order Filter  FilterType=Lowpass  Fo=90  Zeta=0.707  Ts=Ts  Initialize=off  Vac_Init=[0.8 -25 60]  Vdc_Init=-0.4  PlotResponse=off  param1=[1 500 1]
  Gain : Gain
  Iac_SI_to_pu : Gain  Gain=1/Ib/sqrt(2)
  Mux1 : Mux  Inputs=2
  Scope : Scope  NumInputPorts=2
  Sum of Elements : Sum  Inputs=+
  Vac_SI_to_pu1 : Gain  Gain=1/Vb*sqrt(3/2)
  Vac_SI_to_pu2 : Gain  Gain=1/Vdc/2  SampleTime=Ts
  Vdc ctrl : Subsystem
  discrete band pass filter1 : Subsystem  mask(discrete transfer Fcn generator){Fo=frq, adj1=1, inistate=0, Ts=Ts, bodedw=off}
      mask prompts: Fo "F0 (Hz)"; adj1 "adj (1 for no adjustment, larger adj for wider band pass)"; inistate "Initial states"; Ts "Sample time (must be explicite)"; bodedw "draw Bode diagram of filter"
      mask help:
      | This block transfer a continous TF to a discrete TF
      | using Bilinear (Tustin) approximation
      mask init: same as Compare_3level/Rec_VQcontrol1/discrete band pass filter1
  pqctrl : Subsystem
  V_cell_ref : Outport  VectorParamsAs1DForOutWhenUnconnected=off
  wires:
  Constant/1 -> Vdc ctrl/Enable
  Vac_SI_to_pu1/1 -> discrete band pass filter1/1(In1)
  Vac_SI_to_pu2/1 -> Scope/2, Discrete 2nd-Order Filter/1
  Vdc/1 -> Sum of Elements/1
  Discrete 2nd-Order Filter/1 -> Vdc ctrl/1(Vdc)
  Mux1/1 -> pqctrl/3(PQref)
  Demux2/2 -> Mux1/2  "PQref"
  Add1/1 -> Mux1/1
  Vdc ctrl/1(Pcor_lft) -> Gain/1
  Demux2/1 -> Add1/1
  Iac_SI_to_pu/1 -> pqctrl/2(iabcpu)
  Demux1/1 -> Vac_SI_to_pu1/1  "Vabc"
  Demux1/2 -> Iac_SI_to_pu/1  "Iabcpu"
  meas/1 -> Demux1/1
  discrete band pass filter1/1(Out1) -> pqctrl/1(Vabcpu)  "Vabcpu"
  PQref/1 -> Demux2/1  "PQref"
  pqctrl/1(vabc) -> V_cell_ref/1
  Sum of Elements/1 -> Scope/1, Vac_SI_to_pu2/1
  Gain/1 -> Add1/2

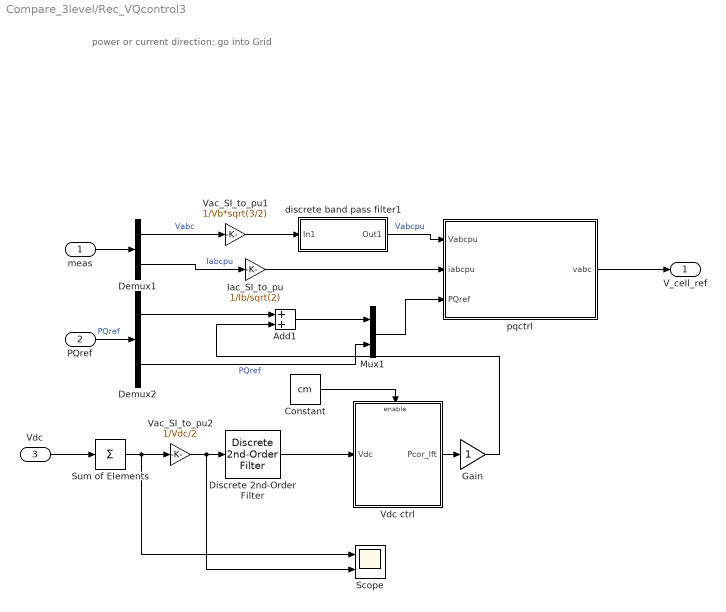
== system Compare_3level/Rec_VQcontrol3 ==
  note: power or current direction: go into Grid
  meas : Inport
  PQref : Inport  Port=2
  Vdc : Inport  Port=3
  Add1 : Sum
  Constant : Constant  Value=cm
  Demux1 : Demux  Outputs=[3 3 ]
  Demux2 : Demux  Outputs=2
  Discrete 2nd-Order Filter : powerlib_extras/Discrete  Control Blocks/Discrete  2nd-Order Filter  FilterType=Lowpass  Fo=90  Zeta=0.707  Ts=Ts  Initialize=off  Vac_Init=[0.8 -25 60]  Vdc_Init=-0.4  PlotResponse=off  param1=[1 500 1]
  Gain : Gain
  Iac_SI_to_pu : Gain  Gain=1/Ib/sqrt(2)
  Mux1 : Mux  Inputs=2
  Scope : Scope  NumInputPorts=2
  Sum of Elements : Sum  Inputs=+
  Vac_SI_to_pu1 : Gain  Gain=1/Vb*sqrt(3/2)
  Vac_SI_to_pu2 : Gain  Gain=1/Vdc/2  SampleTime=Ts
  Vdc ctrl : Subsystem
  discrete band pass filter1 : Subsystem  mask(discrete transfer Fcn generator){Fo=frq, adj1=1, inistate=0, Ts=Ts, bodedw=off}
      mask prompts: Fo "F0 (Hz)"; adj1 "adj (1 for no adjustment, larger adj for wider band pass)"; inistate "Initial states"; Ts "Sample time (must be explicite)"; bodedw "draw Bode diagram of filter"
      mask help:
      | This block transfer a continous TF to a discrete TF
      | using Bilinear (Tustin) approximation
      mask init: same as Compare_3level/Rec_VQcontrol1/discrete band pass filter1
  pqctrl : Subsystem
  V_cell_ref : Outport  VectorParamsAs1DForOutWhenUnconnected=off
  wires:
  Constant/1 -> Vdc ctrl/Enable
  Vac_SI_to_pu1/1 -> discrete band pass filter1/1(In1)
  Vac_SI_to_pu2/1 -> Scope/2, Discrete 2nd-Order Filter/1
  Vdc/1 -> Sum of Elements/1
  Discrete 2nd-Order Filter/1 -> Vdc ctrl/1(Vdc)
  Mux1/1 -> pqctrl/3(PQref)
  Demux2/2 -> Mux1/2  "PQref"
  Add1/1 -> Mux1/1
  Vdc ctrl/1(Pcor_lft) -> Gain/1
  Demux2/1 -> Add1/1
  Iac_SI_to_pu/1 -> pqctrl/2(iabcpu)
  Demux1/1 -> Vac_SI_to_pu1/1  "Vabc"
  Demux1/2 -> Iac_SI_to_pu/1  "Iabcpu"
  meas/1 -> Demux1/1
  discrete band pass filter1/1(Out1) -> pqctrl/1(Vabcpu)  "Vabcpu"
  PQref/1 -> Demux2/1  "PQref"
  pqctrl/1(vabc) -> V_cell_ref/1
  Sum of Elements/1 -> Scope/1, Vac_SI_to_pu2/1
  Gain/1 -> Add1/2

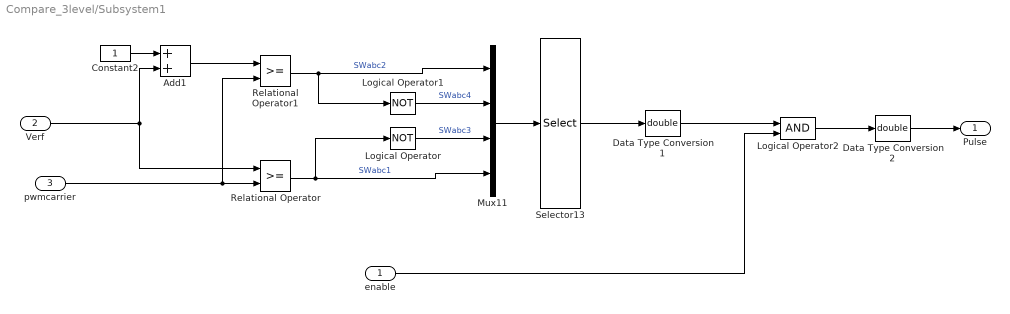
== system Compare_3level/Subsystem1 ==
  enable : Inport
  Verf : Inport  Port=2
  pwmcarrier : Inport  Port=3
  Add1 : Sum
  Constant2 : Constant
  Data Type Conversion1 : DataTypeConversion  OutDataTypeStr=double  SaturateOnIntegerOverflow=off  RndMeth=Floor
  Data Type Conversion2 : DataTypeConversion  OutDataTypeStr=double  SaturateOnIntegerOverflow=off  RndMeth=Floor
  Logical Operator : Logic  Operator=NOT  AllPortsSameDT=off  OutDataTypeStr=boolean
  Logical Operator1 : Logic  Operator=NOT  AllPortsSameDT=off  OutDataTypeStr=boolean
  Logical Operator2 : Logic  AllPortsSameDT=off
  Mux11 : Mux
  Relational Operator : RelationalOperator  OutDataTypeStr=boolean  RndMeth=Simplest  InputSameDT=off
  Relational Operator1 : RelationalOperator  OutDataTypeStr=boolean  RndMeth=Simplest  InputSameDT=off
  Selector13 : Selector  InputPortWidth=12  IndexOptions=Index vector (dialog)  Indices=[10 1 7 4 11 2 8 5 12 3 9 6]  OutputSizes=1
  Pulse : Outport  VectorParamsAs1DForOutWhenUnconnected=off
  wires:
  pwmcarrier/1 -> Relational Operator/2, Relational Operator1/2
  Relational Operator1/1 -> Mux11/1, Logical Operator1/1  "SWabc2"
  Logical Operator/1 -> Mux11/3  "SWabc3"
  Relational Operator/1 -> Logical Operator/1, Mux11/4  "SWabc1"
  Constant2/1 -> Add1/1
  Add1/1 -> Relational Operator1/1
  Verf/1 -> Add1/2, Relational Operator/1
  Selector13/1 -> Data Type Conversion1/1
  Mux11/1 -> Selector13/1
  Logical Operator1/1 -> Mux11/2  "SWabc4"
  Data Type Conversion1/1 -> Logical Operator2/1
  enable/1 -> Logical Operator2/2
  Logical Operator2/1 -> Data Type Conversion2/1
  Data Type Conversion2/1 -> Pulse/1

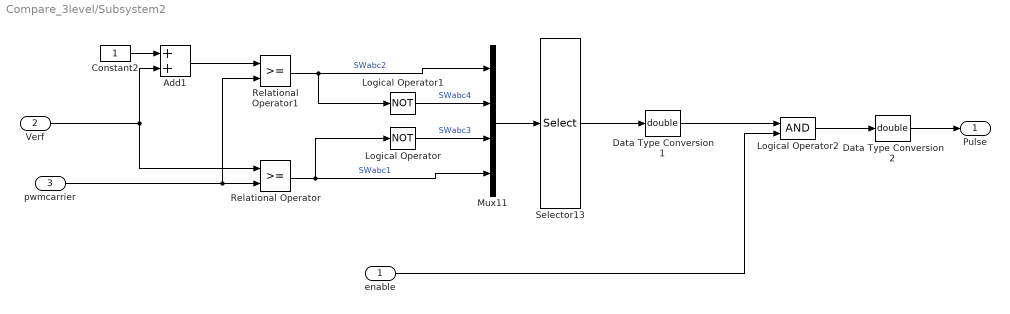
== system Compare_3level/Subsystem2 ==
  enable : Inport
  Verf : Inport  Port=2
  pwmcarrier : Inport  Port=3
  Add1 : Sum
  Constant2 : Constant
  Data Type Conversion1 : DataTypeConversion  OutDataTypeStr=double  SaturateOnIntegerOverflow=off  RndMeth=Floor
  Data Type Conversion2 : DataTypeConversion  OutDataTypeStr=double  SaturateOnIntegerOverflow=off  RndMeth=Floor
  Logical Operator : Logic  Operator=NOT  AllPortsSameDT=off  OutDataTypeStr=boolean
  Logical Operator1 : Logic  Operator=NOT  AllPortsSameDT=off  OutDataTypeStr=boolean
  Logical Operator2 : Logic  AllPortsSameDT=off
  Mux11 : Mux
  Relational Operator : RelationalOperator  OutDataTypeStr=boolean  RndMeth=Simplest  InputSameDT=off
  Relational Operator1 : RelationalOperator  OutDataTypeStr=boolean  RndMeth=Simplest  InputSameDT=off
  Selector13 : Selector  InputPortWidth=12  IndexOptions=Index vector (dialog)  Indices=[10 1 7 4 11 2 8 5 12 3 9 6]  OutputSizes=1
  Pulse : Outport  VectorParamsAs1DForOutWhenUnconnected=off
  wires:
  pwmcarrier/1 -> Relational Operator/2, Relational Operator1/2
  Relational Operator1/1 -> Mux11/1, Logical Operator1/1  "SWabc2"
  Logical Operator/1 -> Mux11/3  "SWabc3"
  Relational Operator/1 -> Logical Operator/1, Mux11/4  "SWabc1"
  Constant2/1 -> Add1/1
  Add1/1 -> Relational Operator1/1
  Verf/1 -> Add1/2, Relational Operator/1
  Selector13/1 -> Data Type Conversion1/1
  Mux11/1 -> Selector13/1
  Logical Operator1/1 -> Mux11/2  "SWabc4"
  Data Type Conversion1/1 -> Logical Operator2/1
  enable/1 -> Logical Operator2/2
  Logical Operator2/1 -> Data Type Conversion2/1
  Data Type Conversion2/1 -> Pulse/1

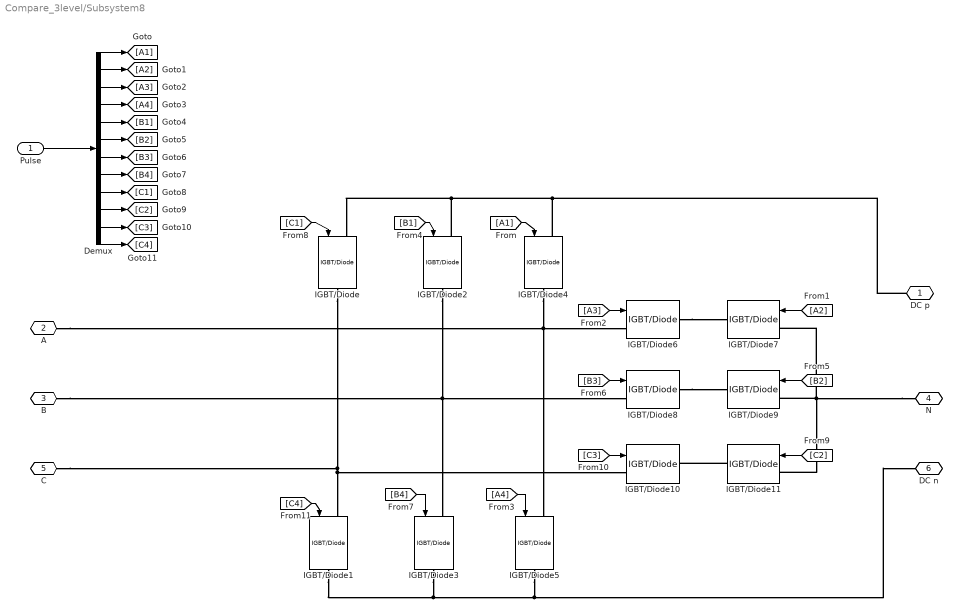
== system Compare_3level/Subsystem8 ==
  Pulse : Inport
  Demux : Demux  Outputs=12
  IGBT/Diode{,1..11} (12 alike) : spsIGBTDiodeLib/IGBT//Diode  Ron=IGBT_Ron  Rs=IGBT_Rs  Cs=IGBT_Cs  Measurements=off
  DC p : PMIOPort  Side=Right
  A : PMIOPort  Port=2  Side=Left
  B : PMIOPort  Port=3  Side=Left
  N : PMIOPort  Port=4  Side=Right
  C : PMIOPort  Port=5  Side=Left
  DC n : PMIOPort  Port=6  Side=Right
  wires:
  [B1] -> IGBT/Diode2/1
  [C1] -> IGBT/Diode/1
  Pulse/1 -> Demux/1
  [C4] -> IGBT/Diode1/1
  [B4] -> IGBT/Diode3/1
  [A4] -> IGBT/Diode5/1
  [A2] -> IGBT/Diode7/1
  [A1] -> IGBT/Diode4/1
  Demux/1 -> [A1]
  Demux/12 -> [C4]
  Demux/2 -> [A2]
  Demux/3 -> [A3]
  Demux/4 -> [A4]
  Demux/5 -> [B1]
  Demux/6 -> [B2]
  Demux/7 -> [B3]
  Demux/8 -> [B4]
  Demux/9 -> [C1]
  Demux/10 -> [C2]
  Demux/11 -> [C3]
  [B2] -> IGBT/Diode9/1
  [C2] -> IGBT/Diode11/1
  [A3] -> IGBT/Diode6/1
  [B3] -> IGBT/Diode8/1
  [C3] -> IGBT/Diode10/1
  connections:
  IGBT/Diode4/RConn1 -- IGBT/Diode6/LConn1 -- IGBT/Diode5/LConn1 -- A/RConn1
  DC p/RConn1 -- IGBT/Diode4/LConn1 -- IGBT/Diode2/LConn1 -- IGBT/Diode/LConn1
  IGBT/Diode6/RConn1 -- IGBT/Diode7/RConn1
  IGBT/Diode2/RConn1 -- IGBT/Diode8/LConn1 -- B/RConn1 -- IGBT/Diode3/LConn1
  IGBT/Diode1/RConn1 -- IGBT/Diode3/RConn1 -- DC n/RConn1 -- IGBT/Diode5/RConn1
  IGBT/Diode8/RConn1 -- IGBT/Diode9/RConn1
  IGBT/Diode11/RConn1 -- IGBT/Diode10/RConn1
  IGBT/Diode/RConn1 -- IGBT/Diode10/LConn1 -- IGBT/Diode1/LConn1 -- C/RConn1
  N/RConn1 -- IGBT/Diode7/LConn1 -- IGBT/Diode11/LConn1 -- IGBT/Diode9/LConn1

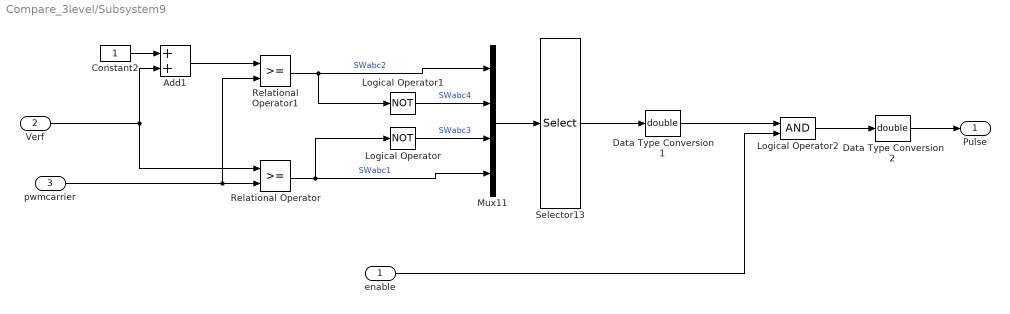
== system Compare_3level/Subsystem9 ==
  enable : Inport
  Verf : Inport  Port=2
  pwmcarrier : Inport  Port=3
  Add1 : Sum
  Constant2 : Constant
  Data Type Conversion1 : DataTypeConversion  OutDataTypeStr=double  SaturateOnIntegerOverflow=off  RndMeth=Floor
  Data Type Conversion2 : DataTypeConversion  OutDataTypeStr=double  SaturateOnIntegerOverflow=off  RndMeth=Floor
  Logical Operator : Logic  Operator=NOT  AllPortsSameDT=off  OutDataTypeStr=boolean
  Logical Operator1 : Logic  Operator=NOT  AllPortsSameDT=off  OutDataTypeStr=boolean
  Logical Operator2 : Logic  AllPortsSameDT=off
  Mux11 : Mux
  Relational Operator : RelationalOperator  OutDataTypeStr=boolean  RndMeth=Simplest  InputSameDT=off
  Relational Operator1 : RelationalOperator  OutDataTypeStr=boolean  RndMeth=Simplest  InputSameDT=off
  Selector13 : Selector  InputPortWidth=12  IndexOptions=Index vector (dialog)  Indices=[10 1 7 4 11 2 8 5 12 3 9 6]  OutputSizes=1
  Pulse : Outport  VectorParamsAs1DForOutWhenUnconnected=off
  wires:
  pwmcarrier/1 -> Relational Operator/2, Relational Operator1/2
  Relational Operator1/1 -> Mux11/1, Logical Operator1/1  "SWabc2"
  Logical Operator/1 -> Mux11/3  "SWabc3"
  Relational Operator/1 -> Logical Operator/1, Mux11/4  "SWabc1"
  Constant2/1 -> Add1/1
  Add1/1 -> Relational Operator1/1
  Verf/1 -> Add1/2, Relational Operator/1
  Selector13/1 -> Data Type Conversion1/1
  Mux11/1 -> Selector13/1
  Logical Operator1/1 -> Mux11/2  "SWabc4"
  Data Type Conversion1/1 -> Logical Operator2/1
  enable/1 -> Logical Operator2/2
  Logical Operator2/1 -> Data Type Conversion2/1
  Data Type Conversion2/1 -> Pulse/1

== system Compare_3level/Rec_VQcontrol1/Vdc ctrl ==
  Vdc : Inport
  Enable : EnablePort  StatesWhenEnabling=reset
  Vdc_ctrler1 : Subsystem
  Pcor_lft : Outport  OutputWhenDisabled=reset  InitialOutput=0  VectorParamsAs1DForOutWhenUnconnected=off
  wires:
  Vdc_ctrler1/1(delP) -> Pcor_lft/1  "Pclft"
  Vdc/1 -> Vdc_ctrler1/1(Vcap)

== system Compare_3level/Rec_VQcontrol1/discrete band pass filter1 ==
  In1 : Inport
  Discrete Transfer Fcn : DiscreteTransferFcn  Numerator=numd  Denominator=dend  InitialStates=inistate  SampleTime=Ts
  Out1 : Outport  VectorParamsAs1DForOutWhenUnconnected=off
  wires:
  Discrete Transfer Fcn/1 -> Out1/1
  In1/1 -> Discrete Transfer Fcn/1

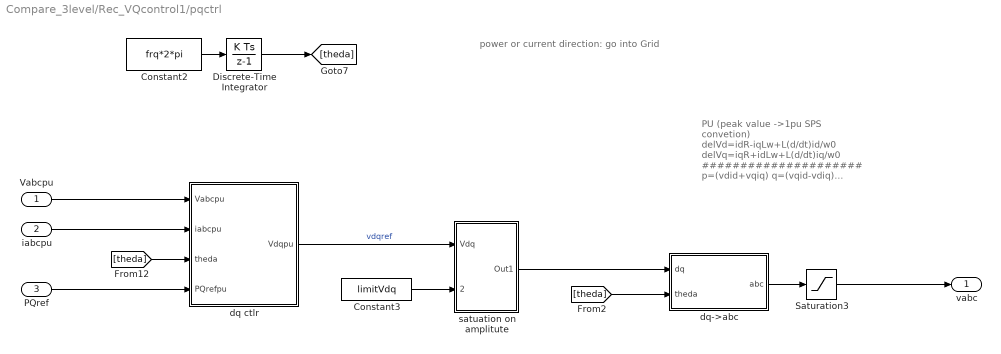
== system Compare_3level/Rec_VQcontrol1/pqctrl ==
  note: PU
      | (peak value ->1pu
      | SPS convetion)
      |
      | delVd=idR-iqLw+L(d/dt)id/w0
      | delVq=iqR+idLw+L(d/dt)iq/w0
      | #####################
      | p=(vdid+vqiq)
      | q=(vqid-vdiq)
      | =>
      | Id=(Vd*P+Vq*Q)/C
      | Iq=(Vq*P-Vd*Q)/C
      | C=Vd^2+Vq^2
  note: power or current direction: go into Grid
  Vabcpu : Inport
  iabcpu : Inport  Port=2
  PQref : Inport  Port=3
  Constant2 : Constant  Value=frq*2*pi
  Constant3 : Constant  Value=limitVdq
  Discrete-Time Integrator : DiscreteIntegrator  SampleTime=Ts  ICPrevOutput=DiscIntNeverNeededParam  ICPrevScaledInput=DiscIntNeverNeededParam
  Saturation3 : Saturate  UpperLimit=Vabc_lim(2)  LowerLimit=Vabc_lim(1)
  dq ctlr : Subsystem
  dq->abc : Subsystem
  "satuation on amplitute " : Subsystem
  vabc : Outport  VectorParamsAs1DForOutWhenUnconnected=off
  wires:
  Saturation3/1 -> vabc/1
  [theda] -> dq->abc/2(theda)
  dq->abc/1(abc) -> Saturation3/1
  Constant3/1 -> "satuation on amplitute "/2(limitVdq)
  "satuation on amplitute "/1(Out1) -> dq->abc/1(dq)
  Constant2/1 -> Discrete-Time Integrator/1
  Discrete-Time Integrator/1 -> [theda]
  [theda] -> dq ctlr/3(theda)
  dq ctlr/1(Vdqpu) -> "satuation on amplitute "/1(Vdq)  "vdqref"
  Vabcpu/1 -> dq ctlr/1(Vabcpu)
  iabcpu/1 -> dq ctlr/2(iabcpu)
  PQref/1 -> dq ctlr/4(PQrefpu)

== system Compare_3level/Rec_VQcontrol2/Vdc ctrl ==
  Vdc : Inport
  Enable : EnablePort  StatesWhenEnabling=reset
  Vdc_ctrler1 : Subsystem
  Pcor_lft : Outport  OutputWhenDisabled=reset  InitialOutput=0  VectorParamsAs1DForOutWhenUnconnected=off
  wires:
  Vdc_ctrler1/1(delP) -> Pcor_lft/1  "Pclft"
  Vdc/1 -> Vdc_ctrler1/1(Vcap)

== system Compare_3level/Rec_VQcontrol2/discrete band pass filter1 ==
  In1 : Inport
  Discrete Transfer Fcn : DiscreteTransferFcn  Numerator=numd  Denominator=dend  InitialStates=inistate  SampleTime=Ts
  Out1 : Outport  VectorParamsAs1DForOutWhenUnconnected=off
  wires:
  Discrete Transfer Fcn/1 -> Out1/1
  In1/1 -> Discrete Transfer Fcn/1

== system Compare_3level/Rec_VQcontrol2/pqctrl ==
  note: PU
      | (peak value ->1pu
      | SPS convetion)
      |
      | delVd=idR-iqLw+L(d/dt)id/w0
      | delVq=iqR+idLw+L(d/dt)iq/w0
      | #####################
      | p=(vdid+vqiq)
      | q=(vqid-vdiq)
      | =>
      | Id=(Vd*P+Vq*Q)/C
      | Iq=(Vq*P-Vd*Q)/C
      | C=Vd^2+Vq^2
  note: power or current direction: go into Grid
  Vabcpu : Inport
  iabcpu : Inport  Port=2
  PQref : Inport  Port=3
  Constant2 : Constant  Value=frq*2*pi
  Constant3 : Constant  Value=limitVdq
  Discrete-Time Integrator : DiscreteIntegrator  SampleTime=Ts  ICPrevOutput=DiscIntNeverNeededParam  ICPrevScaledInput=DiscIntNeverNeededParam
  Saturation3 : Saturate  UpperLimit=Vabc_lim(2)  LowerLimit=Vabc_lim(1)
  dq ctlr : Subsystem
  dq->abc : Subsystem
  "satuation on amplitute " : Subsystem
  vabc : Outport  VectorParamsAs1DForOutWhenUnconnected=off
  wires:
  Saturation3/1 -> vabc/1
  [theda] -> dq->abc/2(theda)
  dq->abc/1(abc) -> Saturation3/1
  Constant3/1 -> "satuation on amplitute "/2(limitVdq)
  "satuation on amplitute "/1(Out1) -> dq->abc/1(dq)
  Constant2/1 -> Discrete-Time Integrator/1
  Discrete-Time Integrator/1 -> [theda]
  [theda] -> dq ctlr/3(theda)
  dq ctlr/1(Vdqpu) -> "satuation on amplitute "/1(Vdq)  "vdqref"
  Vabcpu/1 -> dq ctlr/1(Vabcpu)
  iabcpu/1 -> dq ctlr/2(iabcpu)
  PQref/1 -> dq ctlr/4(PQrefpu)

== system Compare_3level/Rec_VQcontrol3/Vdc ctrl ==
  Vdc : Inport
  Enable : EnablePort  StatesWhenEnabling=reset
  Vdc_ctrler1 : Subsystem
  Pcor_lft : Outport  OutputWhenDisabled=reset  InitialOutput=0  VectorParamsAs1DForOutWhenUnconnected=off
  wires:
  Vdc_ctrler1/1(delP) -> Pcor_lft/1  "Pclft"
  Vdc/1 -> Vdc_ctrler1/1(Vcap)
